simulink library "AP_Connector"  (R2018b)
settings: Solver=VariableStepAuto  StartTime=0.0  StopTime=10.0  RelTol=1e-3

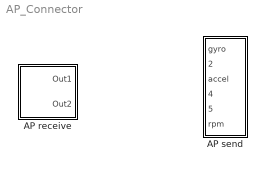
== system AP_Connector ==
  AP receive : Subsystem  AncestorBlock=AP_Conector/AP receive
  AP send : Subsystem  AncestorBlock=AP_Conector/AP send

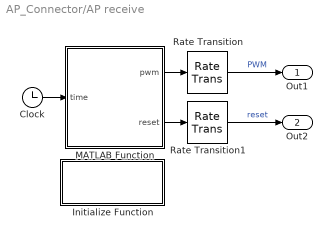
== system AP_Connector/AP receive ==
  Clock : Clock
  Initialize Function : Subsystem  TreatAsAtomicUnit=on
  MATLAB Function : MATLAB Function  TreatAsAtomicUnit=on  SystemSampleTime=1/1000
  Rate Transition : RateTransition
  Rate Transition1 : RateTransition
  Out1 : Outport  VectorParamsAs1DForOutWhenUnconnected=on
  Out2 : Outport  Port=2  VectorParamsAs1DForOutWhenUnconnected=on
  wires:
  Rate Transition1/1 -> Out2/1  "reset"
  MATLAB Function/2(reset) -> Rate Transition1/1
  Clock/1 -> MATLAB Function/1(time)
  MATLAB Function/1(pwm) -> Rate Transition/1
  Rate Transition/1 -> Out1/1  "PWM"

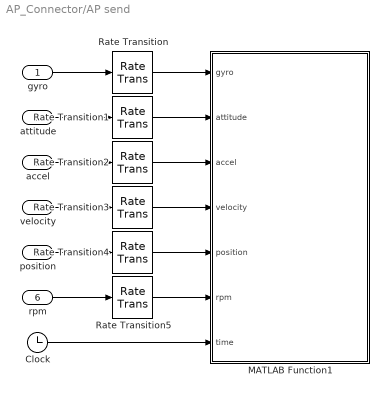
== system AP_Connector/AP send ==
  gyro : Inport
  attitude : Inport  Port=2
  accel : Inport  Port=3
  velocity : Inport  Port=4
  position : Inport  Port=5
  rpm : Inport  Port=6
  Clock : Clock
  MATLAB Function1 : MATLAB Function  TreatAsAtomicUnit=on  SystemSampleTime=1/1000
  Rate Transition{,1..5} (6 alike) : RateTransition
  wires:
  position/1 -> Rate Transition4/1
  velocity/1 -> Rate Transition3/1
  Rate Transition4/1 -> MATLAB Function1/5(position)
  accel/1 -> Rate Transition2/1
  Rate Transition1/1 -> MATLAB Function1/2(attitude)
  Rate Transition2/1 -> MATLAB Function1/3(accel)
  Rate Transition3/1 -> MATLAB Function1/4(velocity)
  Clock/1 -> MATLAB Function1/7(time)
  Rate Transition/1 -> MATLAB Function1/1(gyro)
  gyro/1 -> Rate Transition/1
  attitude/1 -> Rate Transition1/1
  rpm/1 -> Rate Transition5/1
  Rate Transition5/1 -> MATLAB Function1/6(rpm)

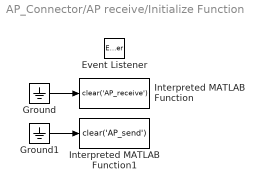
== system AP_Connector/AP receive/Initialize Function ==
  Event Listener : EventListener  DisableCoverage=on  EventName=reset
  Ground : Ground
  Ground1 : Ground
  Interpreted MATLAB Function : MATLABFcn  MATLABFcn=clear('AP_receive')  OutputDimensions=0
  Interpreted MATLAB Function1 : MATLABFcn  MATLABFcn=clear('AP_send')  OutputDimensions=0
  wires:
  Ground/1 -> Interpreted MATLAB Function/1
  Ground1/1 -> Interpreted MATLAB Function1/1

== matlab function AP_Connector/AP receive/MATLAB Function ==
function [pwm, reset]  = fcn(time)
pwm = zeros(16,1); %#ok<PREALL>
reset = false; %#ok<NASGU>
coder.extrinsic('AP_receive')
[pwm, reset] = AP_receive(time);
end

== matlab function AP_Connector/AP send/MATLAB Function1 ==
function fcn(gyro, attitude, accel, velocity, position, rpm, time)
coder.extrinsic('AP_send')
AP_send(gyro, attitude, accel, velocity, position, rpm, time)
end
